simulink model "energy_rigid_wireOnly_quadruped_CPG_BO_fh"  (R2021b)
settings: Solver=ode15s  StartTime=0.0  StopTime=Tf  FixedStep=0.01  MaxStep=0.05  RelTol=0.5  AbsTol=0.5
model workspace (MATLAB code in the model file):
  | %---------------Critical values---------------%
  | angle_amp = pi/4; % Motor rotate amplitude, ref: pi/4
  | rotateCorrectionCoef = 1.158;
  | criticalFn = 2;
  | 
  | %------values for normalization---------------%
  | % values got by running manual gait
  | rotxNormGain = 1/0.1;
  | rotyNormGain = 1/0.05;
  | rotzNormGain = 1/0.1;
  | 
  | vxNormGain = 1/0.2;
  | vyNormGain = 1/0.2;
  | vzNormGain = 1/0.2;
  | 
  | FnNormGain = 1/15;
  | 
  | %--------values for check done---------------%
  | rotDone = pi/6;
  | legBendDone = pi/3; % actuator max bending angle
  | 
  | %---------------Robot parameters-------------%
  | % robot size
  | robot_width = 0.15;
  | robot_length = 0.22;
  | 
  | % floor parameters
  | floor_length = 2;
  | floor_width = 2;
  | 
  | % continuum actuator size
  | L_disk = 0.02944;% Disk side length (m)
  | R_w = L_disk/sqrt(3);
  | thickness_disk = 0.004; % Disk thickness (m)
  | thigh_length = 0.06;
  | R_core = 0.005; % Core radius (m)
  | length_core = 0.008; % Core length (m)
  | R_spool = 0.021; % 0.01944; % radius of the spool
  | spool_height = 0.022+0.015;
  | R_pulley = 1e-3;
  | spool_k = 0;
  | spool_d = 0;
  | hole_d = 4e-3;
  | 
  | % Material property
  | rho_PLA = 1.24e3;
  | rho = 1.19e3; % 1.19e3; % Density (kg/m^3)
  | % use rigid joints
  | Pz_stiff = 135000;
  | Pz_damping = 500*0+2000;
  | S_stiff = 0.0239;
  | S_damping = 7.5e-5;
  | S_low_Bound = -20;
  | S_up_Bound = 20;
  | 
  | R_foot = 0.015; % foot radius (m)
  | 
  | % motor parameter
  | stall_T = 11.2/10; % 11.2 cm*kg, stall torque
  | t_60_deg = 0.2; % 0.09 s
  | V_nomrmal = 6; % corresponding normal voltage
  | Jr = 0.0001; %g*cm^2, robot inertia
  | 
  | % contact force
  | coef_static_friction = 0.315*0+0.6;
  | coef_dynamic_friction = 0.3*0+0.6;
  | crictic_velocity = 0.3; % m/s
  | contact_suf_stiff = 1000*0+750; % N/m
  | contact_suf_damp = 50*0+100; % N/(m/s)
  | contact_region_width = 2e-3; % m
  | spoolOpacity = 0;
  | tendonColor = [0.902 0.902 0.902];
  | tendonOpacity = 0.1;
  | 
  | % If use point masses
  | MMainFrame = 198; % g
  | MServoMotor = 50.55;
  | MMotorSupport = 12.1;
  | MSpool = 9.2;
  | 
  | % Robot total weight about 2 kg
  | MComposateLoad = 200;
  | 
  | MBuck = 40; % x2
  | MPCB_RPi = 141.3;
  | MLiBattery = 120; % x2
  | MPowerBank = 66.5;
  | isLoadVisible = 0.1;
  | 
  | 
  | MThigh = 26.7963;
  | MCore = 0.747699;
  | MDisk = 1.78642;
  | MFoot = 16.8232;
undefined symbols (not defined in the file): A, alpha, alpha_b_gain, alpha_r_gain, DCMotor_K, epsilon, ExtParts, f, init_state, isCheckDone, k, MotorSupport, phase_delay, phi_vec, tau, Tf, TrackStarServo, Ts, WheelCAD, X, Y, Z, z_l_diff, z_l_gain
libraries: sm_lib x311, nesl_utility x81, fl_lib x60, ee_lib x24, slpidlib x12, simulink x11
(part 1 of 16)
settings Model: Creator=Qinglei Ji  LastModifiedBy=kaiget
settings SolverCC: AutoScaleAbsTol=off  MaxConsecutiveZCs=100  MaxConsecutiveMinStep=10  DaesscMode=Fast  ZeroCrossAlgorithm=Adaptive  AutoInsertRateTranBlk=on
settings DebuggingCC: AlgebraicLoopMsg=error  IgnoredZcDiagnostic=none
settings ExplorerConfigSet: InternalSimMechanicsExplorerSettings="<ExplorerConfiguration><canonicalview>default</canonicalview><AnimationSetting><BasePlaybackSpeed>1.0</BasePlaybackSpeed><PlaybackSpeedFactor>1.0</PlaybackSpeedFactor></AnimationSetting><TilePanel><TileInfo><Tiles Columns=\"1\" Count=\"1\" Rows=\"1\"><Column Weight=\"1\"/><Row Weight=\"1\"/><Tile Height=\"1\" Width=\"1\" X=\"0\" Y=\"0\"/></Tiles></TileInfo><SceneInfo><SceneViewer><BGColor><R>0.60000002384185791</R><G>0.60000002384185791</G><B>0.60000002384185791</B></BGColor><Camera><DoPerspective>off</DoPerspective><Position><X>-18.8331461547739707</X><Y>25.880517186070815</Y><Z>26.8100820833696147</Z></Position><Center><X>0.29785977478998571</X><Y>-0.293010908258582892</Y><Z>-0.346783787749327221</Z></Center><Up><X>0.517886432622382209</X><Y>-0.40389178028612327</Y><Z>0.754098848111419029</Z></Up><ViewLimDist>1</ViewLimDist><YLim>0.421333194645766129</YLim><XLim>0.456755011894746488</XLim></Camera></SceneViewer></SceneInfo></TilePanel><MechEditorPanel><Cameras/><GfxPanelCameraMap/><VideoCreator><PlaybackSpeedRatio>1.0</PlaybackSpeedRatio><FrameRate>60</FrameRate><VideoFormat>MPEG-4</VideoFormat><FrameSize>auto</FrameSize></VideoCreator></MechEditorPanel></ExplorerConfiguration>"

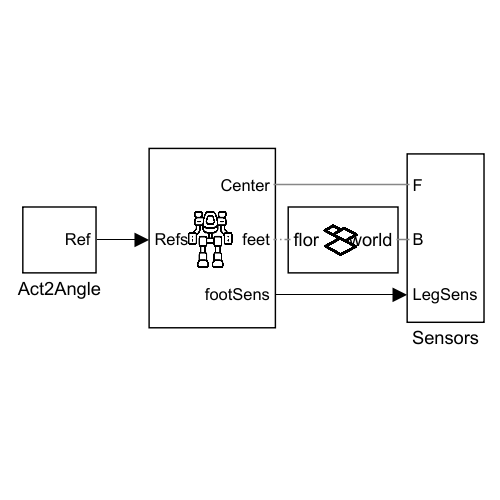
[thumbnail: Simulink's stored preview of the top-level diagram]
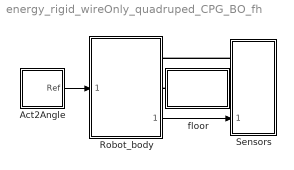
== system energy_rigid_wireOnly_quadruped_CPG_BO_fh ==
  Act2Angle : Subsystem
  Robot_body : Subsystem
      settings: PortSchema="{\"entries\":[{\"content\":{\"sides\":[{\"content\":{\"connectorIds\":[]},\"type\":\"ConnectorPlacement.EquallySpacedRectSide\",\"uuid\":\"6da386a3-61dc-48ac-8951-5f405dad6f0b\"},{\"content\":{\"connectorIds\":[],\"side\":\"RIGHT\"},\"type\":\"ConnectorPlacement.EquallySpacedRectSide\",\"uuid\":\"f31d08fd-e336-4992-a7a1-a5f80310301f\"},{\"content\":{\"connectorIds\":[\"In1\"],\"side\":\"TOP\"},\"type\":\"ConnectorPlacement.EquallySpacedRectSide\",\"uuid\":\"e8d57c74-e878-4fd7-b952-570b3b82c07d\"},{\"content\":{\"connectorIds\":[\"RConn1\",\"RConn2\",\"Out1\"],\"side\":\"BOTTOM\"},\"type\":\"ConnectorPlacement.EquallySpacedRectSide\",\"uuid\":\"5cd044ae-e3eb-4740-b1cb-bb65851cb112\"}]},\"type\":\"ConnectorPlacement.EquallySpacedConnector\",\"uuid\":\"f9915cad-378a-4c2b-ad9c-362eed90ff8c\"}],\"packageUris\":[\"http://schema.mathworks.com/mf0/Connector/R2020b\"],\"version\":\"1.0\"}"
      mask Display: image('$imagefile'); % Use "Edit Image" on toolstrip to change.
  Sensors : Subsystem
      settings: PortSchema="{\"entries\":[{\"content\":{\"sides\":[{\"content\":{\"connectorIds\":[\"LConn1\",\"LConn2\",\"In1\"]},\"type\":\"ConnectorPlacement.EquallySpacedRectSide\",\"uuid\":\"4b5ddd47-03f4-426a-88ee-d6acf531c637\"},{\"content\":{\"connectorIds\":[],\"side\":\"RIGHT\"},\"type\":\"ConnectorPlacement.EquallySpacedRectSide\",\"uuid\":\"f2192e31-fae6-4bce-a663-c668a18a2c9c\"},{\"content\":{\"connectorIds\":[],\"side\":\"TOP\"},\"type\":\"ConnectorPlacement.EquallySpacedRectSide\",\"uuid\":\"20a91eaf-2ad2-4a0d-933a-434c603de7e7\"},{\"content\":{\"connectorIds\":[],\"side\":\"BOTTOM\"},\"type\":\"ConnectorPlacement.EquallySpacedRectSide\",\"uuid\":\"f2757d81-d7c7-43da-8561-08295a517c19\"}]},\"type\":\"ConnectorPlacement.EquallySpacedConnector\",\"uuid\":\"8ce371b8-5669-40c8-963e-855906aef91d\"}],\"packageUris\":[\"http://schema.mathworks.com/mf0/Connector/R2020b\"],\"version\":\"1.0\"}"
  floor : Subsystem
      mask Display: image('$imagefile'); % Use "Edit Image" on toolstrip to change.
  wires:
  Robot_body/1(footSens) -> Sensors/1(LegSens)
  Act2Angle/1(Ref) -> Robot_body/1(motorRefs)
  connections:
  floor/RConn1 -- Robot_body/RConn2
  floor/LConn1 -- Sensors/LConn2
  Sensors/LConn1 -- Robot_body/RConn1

== system energy_rigid_wireOnly_quadruped_CPG_BO_fh/Act2Angle ==
  CPG : Subsystem
  Clock : Clock
  Constant : Constant  Value=zeros(12, 1)
  Human expert : Subsystem  Commented=on
  Manual Switch : ManualSwitch  CurrentSetting=0
  Subsystem : Subsystem
  Switch : Switch  Criteria=u2 > Threshold  Threshold=2
  To Workspace : ToWorkspace  VariableName=action  SaveFormat=Structure  SampleTime=Ts
      settings: Save2DSignal=2-D array (concatenate along first dimension)
  Ref : Outport
  wires:
  Subsystem/1(refs) -> To Workspace/1, Ref/1
  Manual Switch/1 -> Subsystem/1(Acts)  "Acts"
  Human expert/1(Out1) -> Manual Switch/1
  CPG/1(Out2) -> Switch/1
  Clock/1 -> Switch/2
  Constant/1 -> Switch/3
  Switch/1 -> Manual Switch/2

== system energy_rigid_wireOnly_quadruped_CPG_BO_fh/Robot_body ==
  motorRefs : Inport
  6-DOF Joint : sm_lib/Joints/6-DOF Joint  JointMode=Normal  SenseConstraintForce=off  SenseConstraintForceX=off  SenseConstraintForceY=off  SenseConstraintForceZ=off  SenseConstraintTorque=off  SenseConstraintTorqueX=off  SenseConstraintTorqueY=off  SenseConstraintTorqueZ=off  SenseTotalForce=off  SenseTotalForceX=off  SenseTotalForceY=off  SenseTotalForceZ=off  SenseTotalTorque=off  SenseTotalTorqueX=off  SenseTotalTorqueY=off  SenseTotalTorqueZ=off  CompositeWrenchDir=FollowerOnBase  CompositeWrenchFrame=BaseFrame  PxEquilibriumPosition=0  PxEquilibriumPositionUnits=m  PxSpringStiffness=0  PxSpringStiffnessUnits=N/m  PxDampingCoefficient=0  PxDampingCoefficientUnits=N/(m/s)  PxTorqueActuationMode=NoTorque  PxMotionActuationMode=ComputedMotion  PxSensePosition=off  PxSenseVelocity=off  PxSenseAcceleration=off  PxSenseTorqueForce=off  PxSenseLowerLimitTorqueForce=off  PxSenseUpperLimitTorqueForce=off  PxLowerLimitSpecify=off  PxLowerLimitBound=-1  PxLowerLimitBoundUnits=m  PxLowerLimitStiffness=1e6  PxLowerLimitStiffnessUnits=N/m  PxLowerLimitDamping=1e3  PxLowerLimitDampingUnits=N/(m/s)  PxLowerLimitTransitionRegionWidth=1e-4  PxLowerLimitTransitionRegionWidthUnits=m  PxUpperLimitSpecify=off  PxUpperLimitBound=1  PxUpperLimitBoundUnits=m  PxUpperLimitStiffness=1e6  PxUpperLimitStiffnessUnits=N/m  PxUpperLimitDamping=1e3  PxUpperLimitDampingUnits=N/(m/s)  PxUpperLimitTransitionRegionWidth=1e-4  PxUpperLimitTransitionRegionWidthUnits=m  PxPositionTargetSpecify=off  PxPositionTargetPriority=High  PxPositionTargetValue=0  PxPositionTargetValueUnits=m  PxVelocityTargetSpecify=off  PxVelocityTargetPriority=High  PxVelocityTargetValue=0  PxVelocityTargetValueUnits=m/s  PyEquilibriumPosition=0  PyEquilibriumPositionUnits=m  PySpringStiffness=0  PySpringStiffnessUnits=N/m  PyDampingCoefficient=0  PyDampingCoefficientUnits=N/(m/s)  PyTorqueActuationMode=NoTorque  PyMotionActuationMode=ComputedMotion  PySensePosition=off  PySenseVelocity=off  PySenseAcceleration=off  PySenseTorqueForce=off  PySenseLowerLimitTorqueForce=off  PySenseUpperLimitTorqueForce=off  PyLowerLimitSpecify=off  PyLowerLimitBound=-1  PyLowerLimitBoundUnits=m  PyLowerLimitStiffness=1e6  PyLowerLimitStiffnessUnits=N/m  PyLowerLimitDamping=1e3  PyLowerLimitDampingUnits=N/(m/s)  PyLowerLimitTransitionRegionWidth=1e-4  PyLowerLimitTransitionRegionWidthUnits=m  PyUpperLimitSpecify=off  PyUpperLimitBound=1  PyUpperLimitBoundUnits=m  PyUpperLimitStiffness=1e6  PyUpperLimitStiffnessUnits=N/m  PyUpperLimitDamping=1e3  PyUpperLimitDampingUnits=N/(m/s)  PyUpperLimitTransitionRegionWidth=1e-4  PyUpperLimitTransitionRegionWidthUnits=m  PyPositionTargetSpecify=off  PyPositionTargetPriority=High  PyPositionTargetValue=0  PyPositionTargetValueUnits=m  PyVelocityTargetSpecify=off  PyVelocityTargetPriority=High  PyVelocityTargetValue=0  PyVelocityTargetValueUnits=m/s  PzEquilibriumPosition=0  PzEquilibriumPositionUnits=m  PzSpringStiffness=0  PzSpringStiffnessUnits=N/m  PzDampingCoefficient=0  PzDampingCoefficientUnits=N/(m/s)  PzTorqueActuationMode=NoTorque  PzMotionActuationMode=ComputedMotion  PzSensePosition=off  PzSenseVelocity=off  PzSenseAcceleration=off  PzSenseTorqueForce=off  PzSenseLowerLimitTorqueForce=off  PzSenseUpperLimitTorqueForce=off  PzLowerLimitSpecify=off  PzLowerLimitBound=-1  PzLowerLimitBoundUnits=m  PzLowerLimitStiffness=1e6  PzLowerLimitStiffnessUnits=N/m  PzLowerLimitDamping=1e3  PzLowerLimitDampingUnits=N/(m/s)  PzLowerLimitTransitionRegionWidth=1e-4  PzLowerLimitTransitionRegionWidthUnits=m  PzUpperLimitSpecify=off  PzUpperLimitBound=1  PzUpperLimitBoundUnits=m  PzUpperLimitStiffness=1e6  PzUpperLimitStiffnessUnits=N/m  PzUpperLimitDamping=1e3  PzUpperLimitDampingUnits=N/(m/s)  PzUpperLimitTransitionRegionWidth=1e-4  PzUpperLimitTransitionRegionWidthUnits=m  PzPositionTargetSpecify=off  PzPositionTargetPriority=High  PzPositionTargetValue=0  PzPositionTargetValueUnits=m  PzVelocityTargetSpecify=off  PzVelocityTargetPriority=High  PzVelocityTargetValue=0  PzVelocityTargetValueUnits=m/s  SphDefPosRotationMethod=None  SphDefPosRotationAngleUnits=deg  SphDefPosRotationStandardAxis=+Z  SphDefPosRotationAngle=0.0  SphDefPosRotationArbitraryAxis=[0 0 1]  SphDefPosFollAlignAxisA=+X  SphDefPosBaseAlignAxisA=+Y  SphDefPosFollAlignAxisB=+Y  SphDefPosBaseAlignAxisB=+Z  SphDefPosRotationSequenceAxes=FollowerAxes  SphDefPosRotationSequence=XYX  SphDefPosRotationSequenceAngles=[0 0 0]  SphDefPosRotationSequenceAnglesUnits=deg  SphDefPosRotationMatrix=[1 0 0; 0 1 0; 0 0 1]  SphEqPosRotationMethod=None  SphEqPosRotationAngleUnits=deg  SphEqPosRotationStandardAxis=+Z  SphEqPosRotationAngle=0.0  SphEqPosRotationArbitraryAxis=[0 0 1]  SphEqPosFollAlignAxisA=+X  SphEqPosBaseAlignAxisA=+Y  SphEqPosFollAlignAxisB=+Y  SphEqPosBaseAlignAxisB=+Z  SphEqPosRotationSequenceAxes=FollowerAxes  SphEqPosRotationSequence=XYX  SphEqPosRotationSequenceAngles=[0 0 0]  SphEqPosRotationSequenceAnglesUnits=deg  SphEqPosRotationMatrix=[1 0 0; 0 1 0; 0 0 1]  SphSpringStiffness=0  SphSpringStiffnessUnits=N*m/deg  SphDampingCoefficient=0  SphDampingCoefficientUnits=N*m/(deg/s)  SphActuateTorqueX=off  SphActuateTorqueY=off  SphActuateTorqueZ=off  SphActuateTorque=off  SphTorqueActuationMode=NoTorque  SphMotionActuationMode=ComputedMotion  SphActuationFrame=BaseFrame  SphSensePosition=off  SphSenseVelocityX=off  SphSenseVelocityY=off  SphSenseVelocityZ=off  SphSenseVelocity=off  SphSenseAccelerationX=off  SphSenseAccelerationY=off  SphSenseAccelerationZ=off  SphSenseAcceleration=off  SphSenseTorqueX=off  SphSenseTorqueY=off  SphSenseTorqueZ=off  SphSenseTorqueForce=off  SphSenseLowerLimitTorqueMag=off  SphSenseUpperLimitTorqueMag=off  SphSensingFrame=BaseFrame  SphLowerLimitSpecify=off  SphLowerLimitBound=15  SphLowerLimitBoundUnits=deg  SphLowerLimitStiffness=1e4  SphLowerLimitStiffnessUnits=N*m/deg  SphLowerLimitDamping=10  SphLowerLimitDampingUnits=N*m/(deg/s)  SphLowerLimitTransitionRegionWidth=0.1  SphLowerLimitTransitionRegionWidthUnits=deg  SphUpperLimitSpecify=off  SphUpperLimitBound=45  SphUpperLimitBoundUnits=deg  SphUpperLimitStiffness=1e4  SphUpperLimitStiffnessUnits=N*m/deg  SphUpperLimitDamping=10  SphUpperLimitDampingUnits=N*m/(deg/s)  SphUpperLimitTransitionRegionWidth=0.1  SphUpperLimitTransitionRegionWidthUnits=deg  SphPositionTargetRotationMethod=None  SphPositionTargetRotationAngleUnits=deg  SphPositionTargetRotationStandardAxis=+Z  SphPositionTargetRotationAngle=0.0  SphPositionTargetRotationArbitraryAxis=[0 0 1]  SphPositionTargetFollAlignAxisA=+X  SphPositionTargetBaseAlignAxisA=+Y  SphPositionTargetFollAlignAxisB=+Y  SphPositionTargetBaseAlignAxisB=+Z  SphPositionTargetRotationSequenceAxes=FollowerAxes  SphPositionTargetRotationSequence=XYX  SphPositionTargetRotationSequenceAngles=[0 0 0]  SphPositionTargetRotationSequenceAnglesUnits=deg  SphPositionTargetRotationMatrix=[1 0 0; 0 1 0; 0 0 1]  SphPositionTargetSpecify=off  SphPositionTargetPriority=High  SphVelocityTargetValue=[0 0 0]  SphVelocityTargetValueUnits=deg/s  SphVelocityTargetSpecify=off  SphVelocityTargetPriority=High  SphVelocityTargetInFollowerFrame=on
  Bus Creator : BusCreator  Inputs=12
  Demux : Demux
  FL : Subsystem
  FR : Subsystem
  FootFL : Subsystem
      settings: PortSchema="{\"entries\":[{\"content\":{\"sides\":[{\"content\":{\"connectorIds\":[\"LConn1\",\"Out1\"]},\"type\":\"ConnectorPlacement.EquallySpacedRectSide\",\"uuid\":\"0bb1f20c-4b5e-487a-8abf-3e1f2fef015b\"},{\"content\":{\"connectorIds\":[\"RConn1\"],\"side\":\"RIGHT\"},\"type\":\"ConnectorPlacement.EquallySpacedRectSide\",\"uuid\":\"5d13e6ab-8a90-4d8e-960d-d3cf2c1ae97d\"},{\"content\":{\"connectorIds\":[],\"side\":\"TOP\"},\"type\":\"ConnectorPlacement.EquallySpacedRectSide\",\"uuid\":\"95bd9573-7fea-4bcb-a448-c8ab92610e8b\"},{\"content\":{\"connectorIds\":[],\"side\":\"BOTTOM\"},\"type\":\"ConnectorPlacement.EquallySpacedRectSide\",\"uuid\":\"976c40b0-0fd4-4a26-8e09-25e540e36d50\"}]},\"type\":\"ConnectorPlacement.EquallySpacedConnector\",\"uuid\":\"5d9c26bf-393c-4096-afaf-0ed92cf9ce69\"}],\"packageUris\":[\"http://schema.mathworks.com/mf0/Connector/R2020b\"],\"version\":\"1.0\"}"
  FootFR : Subsystem
      settings: PortSchema="{\"entries\":[{\"content\":{\"sides\":[{\"content\":{\"connectorIds\":[\"LConn1\",\"Out1\"]},\"type\":\"ConnectorPlacement.EquallySpacedRectSide\",\"uuid\":\"0bb1f20c-4b5e-487a-8abf-3e1f2fef015b\"},{\"content\":{\"connectorIds\":[\"RConn1\"],\"side\":\"RIGHT\"},\"type\":\"ConnectorPlacement.EquallySpacedRectSide\",\"uuid\":\"5d13e6ab-8a90-4d8e-960d-d3cf2c1ae97d\"},{\"content\":{\"connectorIds\":[],\"side\":\"TOP\"},\"type\":\"ConnectorPlacement.EquallySpacedRectSide\",\"uuid\":\"95bd9573-7fea-4bcb-a448-c8ab92610e8b\"},{\"content\":{\"connectorIds\":[],\"side\":\"BOTTOM\"},\"type\":\"ConnectorPlacement.EquallySpacedRectSide\",\"uuid\":\"976c40b0-0fd4-4a26-8e09-25e540e36d50\"}]},\"type\":\"ConnectorPlacement.EquallySpacedConnector\",\"uuid\":\"5d9c26bf-393c-4096-afaf-0ed92cf9ce69\"}],\"packageUris\":[\"http://schema.mathworks.com/mf0/Connector/R2020b\"],\"version\":\"1.0\"}"
  FootRL : Subsystem
      settings: PortSchema="{\"entries\":[{\"content\":{\"sides\":[{\"content\":{\"connectorIds\":[\"LConn1\",\"Out1\"]},\"type\":\"ConnectorPlacement.EquallySpacedRectSide\",\"uuid\":\"0bb1f20c-4b5e-487a-8abf-3e1f2fef015b\"},{\"content\":{\"connectorIds\":[\"RConn1\"],\"side\":\"RIGHT\"},\"type\":\"ConnectorPlacement.EquallySpacedRectSide\",\"uuid\":\"5d13e6ab-8a90-4d8e-960d-d3cf2c1ae97d\"},{\"content\":{\"connectorIds\":[],\"side\":\"TOP\"},\"type\":\"ConnectorPlacement.EquallySpacedRectSide\",\"uuid\":\"95bd9573-7fea-4bcb-a448-c8ab92610e8b\"},{\"content\":{\"connectorIds\":[],\"side\":\"BOTTOM\"},\"type\":\"ConnectorPlacement.EquallySpacedRectSide\",\"uuid\":\"976c40b0-0fd4-4a26-8e09-25e540e36d50\"}]},\"type\":\"ConnectorPlacement.EquallySpacedConnector\",\"uuid\":\"5d9c26bf-393c-4096-afaf-0ed92cf9ce69\"}],\"packageUris\":[\"http://schema.mathworks.com/mf0/Connector/R2020b\"],\"version\":\"1.0\"}"
  FootRR : Subsystem
      settings: PortSchema="{\"entries\":[{\"content\":{\"sides\":[{\"content\":{\"connectorIds\":[\"LConn1\",\"Out1\"]},\"type\":\"ConnectorPlacement.EquallySpacedRectSide\",\"uuid\":\"0bb1f20c-4b5e-487a-8abf-3e1f2fef015b\"},{\"content\":{\"connectorIds\":[\"RConn1\"],\"side\":\"RIGHT\"},\"type\":\"ConnectorPlacement.EquallySpacedRectSide\",\"uuid\":\"5d13e6ab-8a90-4d8e-960d-d3cf2c1ae97d\"},{\"content\":{\"connectorIds\":[],\"side\":\"TOP\"},\"type\":\"ConnectorPlacement.EquallySpacedRectSide\",\"uuid\":\"95bd9573-7fea-4bcb-a448-c8ab92610e8b\"},{\"content\":{\"connectorIds\":[],\"side\":\"BOTTOM\"},\"type\":\"ConnectorPlacement.EquallySpacedRectSide\",\"uuid\":\"976c40b0-0fd4-4a26-8e09-25e540e36d50\"}]},\"type\":\"ConnectorPlacement.EquallySpacedConnector\",\"uuid\":\"5d9c26bf-393c-4096-afaf-0ed92cf9ce69\"}],\"packageUris\":[\"http://schema.mathworks.com/mf0/Connector/R2020b\"],\"version\":\"1.0\"}"
  RL : Subsystem
  RR : Subsystem
  Rigid Transform : sm_lib/Frames and Transforms/Rigid Transform  TranslationMethod=None  TranslationStandardOffset=0.1  TranslationLengthUnit=m  TranslationStandardAxis=+Z  TranslationCartesianOffset=[0 0 0]  TranslationROffset=0  TranslationROffsetUnits=m  TranslationZOffset=0  TranslationZOffsetUnits=m  TranslationThetaOffset=0  TranslationThetaOffsetUnits=deg  RotationMethod=StandardAxis  RotationAngleUnits=deg  RotationStandardAxis=-Z  RotationAngle=90  RotationArbitraryAxis=[0 0 1]  FollAlignAxisA=+X  BaseAlignAxisA=+Z  FollAlignAxisB=+Y  BaseAlignAxisB=+Z  RotationSequenceAxes=FollowerAxes  RotationSequence=XYX  RotationSequenceAngles=[0 0 0]  RotationSequenceAnglesUnits=deg  RotationMatrix=[1 0 0; 0 1 0; 0 0 1]
  Rigid Transform1 : sm_lib/Frames and Transforms/Rigid Transform  TranslationMethod=None  TranslationStandardOffset=0.1  TranslationLengthUnit=m  TranslationStandardAxis=+Z  TranslationCartesianOffset=[0 0 0]  TranslationROffset=0  TranslationROffsetUnits=m  TranslationZOffset=0  TranslationZOffsetUnits=m  TranslationThetaOffset=0  TranslationThetaOffsetUnits=deg  RotationMethod=StandardAxis  RotationAngleUnits=deg  RotationStandardAxis=+Z  RotationAngle=90  RotationArbitraryAxis=[0 0 1]  FollAlignAxisA=+X  BaseAlignAxisA=+Z  FollAlignAxisB=+Y  BaseAlignAxisB=+Z  RotationSequenceAxes=FollowerAxes  RotationSequence=XYX  RotationSequenceAngles=[0 0 0]  RotationSequenceAnglesUnits=deg  RotationMatrix=[1 0 0; 0 1 0; 0 0 1]
  Rigid Transform2 : sm_lib/Frames and Transforms/Rigid Transform  TranslationMethod=Cartesian  TranslationStandardOffset=0  TranslationLengthUnit=m  TranslationStandardAxis=+Z  TranslationCartesianOffset=[robot_length/2 -robot_width/2 0]  TranslationROffset=0  TranslationROffsetUnits=m  TranslationZOffset=0  TranslationZOffsetUnits=m  TranslationThetaOffset=0  TranslationThetaOffsetUnits=deg  RotationMethod=None  RotationAngleUnits=deg  RotationStandardAxis=+Z  RotationAngle=0.0  RotationArbitraryAxis=[0 0 1]  FollAlignAxisA=+X  BaseAlignAxisA=+Y  FollAlignAxisB=+Y  BaseAlignAxisB=+Z  RotationSequenceAxes=FollowerAxes  RotationSequence=XYX  RotationSequenceAngles=[0 0 0]  RotationSequenceAnglesUnits=deg  RotationMatrix=[1 0 0; 0 1 0; 0 0 1]
  Rigid Transform3 : sm_lib/Frames and Transforms/Rigid Transform  TranslationMethod=Cartesian  TranslationStandardOffset=0  TranslationLengthUnit=m  TranslationStandardAxis=+Z  TranslationCartesianOffset=[robot_length/2 robot_width/2 0]  TranslationROffset=0  TranslationROffsetUnits=m  TranslationZOffset=0  TranslationZOffsetUnits=m  TranslationThetaOffset=0  TranslationThetaOffsetUnits=deg  RotationMethod=None  RotationAngleUnits=deg  RotationStandardAxis=+Z  RotationAngle=0.0  RotationArbitraryAxis=[0 0 1]  FollAlignAxisA=+X  BaseAlignAxisA=+Y  FollAlignAxisB=+Y  BaseAlignAxisB=+Z  RotationSequenceAxes=FollowerAxes  RotationSequence=XYX  RotationSequenceAngles=[0 0 0]  RotationSequenceAnglesUnits=deg  RotationMatrix=[1 0 0; 0 1 0; 0 0 1]
  Rigid Transform4 : sm_lib/Frames and Transforms/Rigid Transform  TranslationMethod=Cartesian  TranslationStandardOffset=0  TranslationLengthUnit=m  TranslationStandardAxis=+Z  TranslationCartesianOffset=[-robot_length/2 -robot_width/2 0]  TranslationROffset=0  TranslationROffsetUnits=m  TranslationZOffset=0  TranslationZOffsetUnits=m  TranslationThetaOffset=0  TranslationThetaOffsetUnits=deg  RotationMethod=None  RotationAngleUnits=deg  RotationStandardAxis=+Z  RotationAngle=0.0  RotationArbitraryAxis=[0 0 1]  FollAlignAxisA=+X  BaseAlignAxisA=+Y  FollAlignAxisB=+Y  BaseAlignAxisB=+Z  RotationSequenceAxes=FollowerAxes  RotationSequence=XYX  RotationSequenceAngles=[0 0 0]  RotationSequenceAnglesUnits=deg  RotationMatrix=[1 0 0; 0 1 0; 0 0 1]
  Rigid Transform5 : sm_lib/Frames and Transforms/Rigid Transform  TranslationMethod=Cartesian  TranslationStandardOffset=0  TranslationLengthUnit=m  TranslationStandardAxis=+Z  TranslationCartesianOffset=[-robot_length/2 robot_width/2 0]  TranslationROffset=0  TranslationROffsetUnits=m  TranslationZOffset=0  TranslationZOffsetUnits=m  TranslationThetaOffset=0  TranslationThetaOffsetUnits=deg  RotationMethod=None  RotationAngleUnits=deg  RotationStandardAxis=+Z  RotationAngle=0.0  RotationArbitraryAxis=[0 0 1]  FollAlignAxisA=+X  BaseAlignAxisA=+Y  FollAlignAxisB=+Y  BaseAlignAxisB=+Z  RotationSequenceAxes=FollowerAxes  RotationSequence=XYX  RotationSequenceAngles=[0 0 0]  RotationSequenceAnglesUnits=deg  RotationMatrix=[1 0 0; 0 1 0; 0 0 1]
  Rigid Transform9 : sm_lib/Frames and Transforms/Rigid Transform  TranslationMethod=Cartesian  TranslationStandardOffset=0  TranslationLengthUnit=m  TranslationStandardAxis=+Z  TranslationCartesianOffset=[0 0 0.155]  TranslationROffset=0  TranslationROffsetUnits=m  TranslationZOffset=0  TranslationZOffsetUnits=m  TranslationThetaOffset=0  TranslationThetaOffsetUnits=deg  RotationMethod=StandardAxis  RotationAngleUnits=deg  RotationStandardAxis=+Y  RotationAngle=0  RotationArbitraryAxis=[0 0 1]  FollAlignAxisA=+X  BaseAlignAxisA=+Y  FollAlignAxisB=+Y  BaseAlignAxisB=+Z  RotationSequenceAxes=FollowerAxes  RotationSequence=XYX  RotationSequenceAngles=[0 0 0]  RotationSequenceAnglesUnits=deg  RotationMatrix=[1 0 0; 0 1 0; 0 0 1]
  StructureDisk : Subsystem
      settings: PortSchema="{\"entries\":[{\"content\":{\"sides\":[{\"content\":{\"connectorIds\":[]},\"type\":\"ConnectorPlacement.EquallySpacedRectSide\",\"uuid\":\"983b4593-33f8-4f05-8496-f6a680e0506a\"},{\"content\":{\"connectorIds\":[\"RConn1\"],\"side\":\"RIGHT\"},\"type\":\"ConnectorPlacement.EquallySpacedRectSide\",\"uuid\":\"dd1cb835-99ed-40eb-9457-9a76e9b19610\"},{\"content\":{\"connectorIds\":[\"LConn1\"],\"side\":\"TOP\"},\"type\":\"ConnectorPlacement.EquallySpacedRectSide\",\"uuid\":\"c15c4885-45e6-4882-9e3a-df9802ff439f\"}]},\"type\":\"ConnectorPlacement.EquallySpacedConnector\",\"uuid\":\"19826241-0a68-4e2d-83d2-fcb027292ea7\"}],\"packageUris\":[\"http://schema.mathworks.com/mf0/Connector/R2020b\"],\"version\":\"1.0\"}"
      mask DialogControl DescTextVar Prompt: StructureDisk.png
      mask Display: image('$imagefile'); % Use "Edit Image" on toolstrip to change.
  World Frame : sm_lib/Frames and Transforms/World Frame
  sensFL : Subsystem
      settings: PortSchema="{\"entries\":[{\"content\":{\"sides\":[{\"content\":{\"connectorIds\":[]},\"type\":\"ConnectorPlacement.EquallySpacedRectSide\",\"uuid\":\"bd83465d-2bef-45ec-b31a-ccd96dc04922\"},{\"content\":{\"connectorIds\":[],\"side\":\"RIGHT\"},\"type\":\"ConnectorPlacement.EquallySpacedRectSide\",\"uuid\":\"7d39c37e-7359-45a9-8850-f640f6442332\"},{\"content\":{\"connectorIds\":[\"LConn1\"],\"side\":\"TOP\"},\"type\":\"ConnectorPlacement.EquallySpacedRectSide\",\"uuid\":\"9171d6ae-b8cc-4ed2-b32d-fb0addba6640\"},{\"content\":{\"connectorIds\":[\"Out1\",\"RConn1\"],\"side\":\"BOTTOM\"},\"type\":\"ConnectorPlacement.EquallySpacedRectSide\",\"uuid\":\"6d61618f-1cbe-4c91-8d9a-cf1c63ddd154\"}]},\"type\":\"ConnectorPlacement.EquallySpacedConnector\",\"uuid\":\"3aecd3e6-ec94-4a95-ad20-92352af1806b\"}],\"packageUris\":[\"http://schema.mathworks.com/mf0/Connector/R2020b\"],\"version\":\"1.0\"}"
  sensFR : Subsystem
      settings: PortSchema="{\"entries\":[{\"content\":{\"sides\":[{\"content\":{\"connectorIds\":[]},\"type\":\"ConnectorPlacement.EquallySpacedRectSide\",\"uuid\":\"bd83465d-2bef-45ec-b31a-ccd96dc04922\"},{\"content\":{\"connectorIds\":[],\"side\":\"RIGHT\"},\"type\":\"ConnectorPlacement.EquallySpacedRectSide\",\"uuid\":\"7d39c37e-7359-45a9-8850-f640f6442332\"},{\"content\":{\"connectorIds\":[\"LConn1\"],\"side\":\"TOP\"},\"type\":\"ConnectorPlacement.EquallySpacedRectSide\",\"uuid\":\"9171d6ae-b8cc-4ed2-b32d-fb0addba6640\"},{\"content\":{\"connectorIds\":[\"Out1\",\"RConn1\"],\"side\":\"BOTTOM\"},\"type\":\"ConnectorPlacement.EquallySpacedRectSide\",\"uuid\":\"6d61618f-1cbe-4c91-8d9a-cf1c63ddd154\"}]},\"type\":\"ConnectorPlacement.EquallySpacedConnector\",\"uuid\":\"3aecd3e6-ec94-4a95-ad20-92352af1806b\"}],\"packageUris\":[\"http://schema.mathworks.com/mf0/Connector/R2020b\"],\"version\":\"1.0\"}"
  sensRL : Subsystem
      settings: PortSchema="{\"entries\":[{\"content\":{\"sides\":[{\"content\":{\"connectorIds\":[]},\"type\":\"ConnectorPlacement.EquallySpacedRectSide\",\"uuid\":\"bd83465d-2bef-45ec-b31a-ccd96dc04922\"},{\"content\":{\"connectorIds\":[],\"side\":\"RIGHT\"},\"type\":\"ConnectorPlacement.EquallySpacedRectSide\",\"uuid\":\"7d39c37e-7359-45a9-8850-f640f6442332\"},{\"content\":{\"connectorIds\":[\"LConn1\"],\"side\":\"TOP\"},\"type\":\"ConnectorPlacement.EquallySpacedRectSide\",\"uuid\":\"9171d6ae-b8cc-4ed2-b32d-fb0addba6640\"},{\"content\":{\"connectorIds\":[\"Out1\",\"RConn1\"],\"side\":\"BOTTOM\"},\"type\":\"ConnectorPlacement.EquallySpacedRectSide\",\"uuid\":\"6d61618f-1cbe-4c91-8d9a-cf1c63ddd154\"}]},\"type\":\"ConnectorPlacement.EquallySpacedConnector\",\"uuid\":\"3aecd3e6-ec94-4a95-ad20-92352af1806b\"}],\"packageUris\":[\"http://schema.mathworks.com/mf0/Connector/R2020b\"],\"version\":\"1.0\"}"
  sensRR : Subsystem
      settings: PortSchema="{\"entries\":[{\"content\":{\"sides\":[{\"content\":{\"connectorIds\":[]},\"type\":\"ConnectorPlacement.EquallySpacedRectSide\",\"uuid\":\"bd83465d-2bef-45ec-b31a-ccd96dc04922\"},{\"content\":{\"connectorIds\":[],\"side\":\"RIGHT\"},\"type\":\"ConnectorPlacement.EquallySpacedRectSide\",\"uuid\":\"7d39c37e-7359-45a9-8850-f640f6442332\"},{\"content\":{\"connectorIds\":[\"LConn1\"],\"side\":\"TOP\"},\"type\":\"ConnectorPlacement.EquallySpacedRectSide\",\"uuid\":\"9171d6ae-b8cc-4ed2-b32d-fb0addba6640\"},{\"content\":{\"connectorIds\":[\"Out1\",\"RConn1\"],\"side\":\"BOTTOM\"},\"type\":\"ConnectorPlacement.EquallySpacedRectSide\",\"uuid\":\"6d61618f-1cbe-4c91-8d9a-cf1c63ddd154\"}]},\"type\":\"ConnectorPlacement.EquallySpacedConnector\",\"uuid\":\"3aecd3e6-ec94-4a95-ad20-92352af1806b\"}],\"packageUris\":[\"http://schema.mathworks.com/mf0/Connector/R2020b\"],\"version\":\"1.0\"}"
  Center : PMIOPort  Side=Right
  feet : PMIOPort  Port=2  Side=Right
  footSens : Outport
  wires:
  [refFR] -> FR/1(In1)  "refFR"
  [refFL] -> FL/1(In1)  "refFL"
  [refRR] -> RR/1(In1)  "refRR"
  [refRL] -> RL/1(In1)  "refRL"
  Bus Creator/1 -> footSens/1
  FootFR/1(sensor) -> Bus Creator/2
  FootFL/1(sensor) -> Bus Creator/5
  FootRL/1(sensor) -> Bus Creator/8
  FootRR/1(sensor) -> Bus Creator/11
  sensFR/1(bend) -> Bus Creator/3
  sensFL/1(bend) -> Bus Creator/6
  sensRL/1(bend) -> Bus Creator/9
  sensRR/1(bend) -> Bus Creator/12
  Demux/1 -> [refFR]
  Demux/2 -> [refFL]
  Demux/3 -> [refRL]
  Demux/4 -> [refRR]
  motorRefs/1 -> Demux/1  "Refs"
  FR/1(powers) -> Bus Creator/1  "powerFR"
  FL/1(powers) -> Bus Creator/4  "powerFL"
  RL/1(powers) -> Bus Creator/7  "powerRL"
  RR/1(powers) -> Bus Creator/10  "powerRR"
  connections:
  sensFL/LConn1 -- FL/LConn1 -- Rigid Transform4/LConn1
  sensRR/LConn1 -- RR/LConn1 -- Rigid Transform3/LConn1
  sensRL/LConn1 -- RL/LConn1 -- Rigid Transform2/LConn1
  FootFR/LConn1 -- FootFL/LConn1 -- feet/RConn1 -- FootRR/LConn1 -- FootRL/LConn1
  sensFL/RConn1 -- FL/RConn1 -- FootFL/RConn1
  sensRL/RConn1 -- RL/RConn1 -- FootRL/RConn1
  sensRR/RConn1 -- RR/RConn1 -- FootRR/RConn1
  Rigid Transform2/RConn1 -- Rigid Transform3/RConn1 -- Rigid Transform1/LConn1 -- Rigid Transform5/RConn1 -- Rigid Transform4/RConn1
  Rigid Transform/LConn1 -- StructureDisk/LConn1
  StructureDisk/RConn1 -- Rigid Transform1/RConn1
  Rigid Transform/RConn1 -- 6-DOF Joint/RConn1 -- Center/RConn1
  FR/LConn1 -- sensFR/LConn1 -- Rigid Transform5/LConn1
  FR/RConn1 -- FootFR/RConn1 -- sensFR/RConn1
  Rigid Transform9/RConn1 -- 6-DOF Joint/LConn1
  Rigid Transform9/LConn1 -- World Frame/RConn1

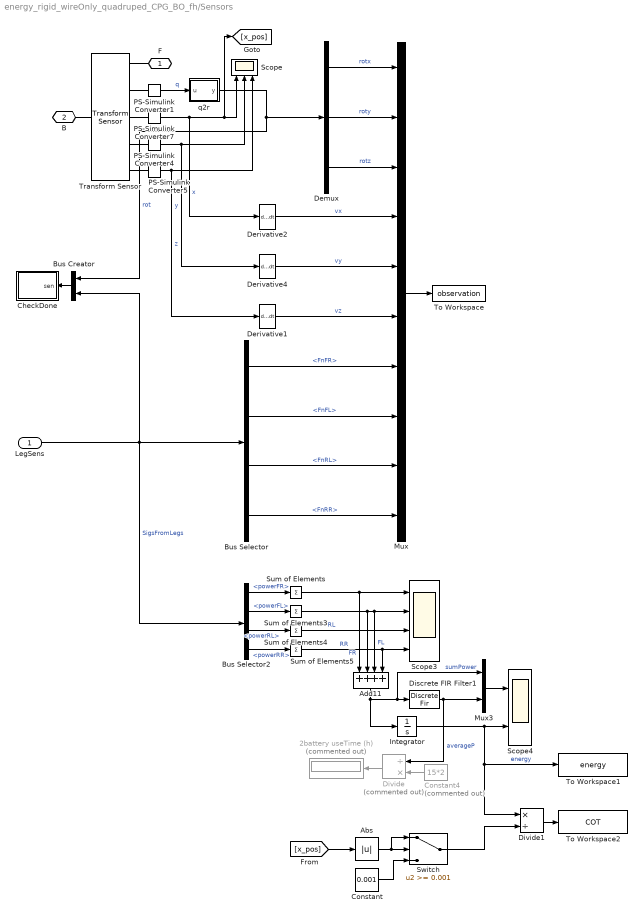
== system energy_rigid_wireOnly_quadruped_CPG_BO_fh/Sensors ==
  LegSens : Inport
  2battery useTime (h) : Display  Commented=on
  Abs : Abs
  Add11 : Sum  Inputs=++++
  Bus Creator : BusCreator  Inputs=2
  Bus Selector : BusSelector  OutputSignals=FnFR,FnFL,FnRL,FnRR
  Bus Selector2 : BusSelector  OutputSignals=powerFR,powerFL,powerRL,powerRR
  CheckDone : Subsystem
  Constant : Constant  Value=0.001
  Constant4 : Constant  Commented=on  Value=15*2
  Demux : Demux  Outputs=3
  Derivative1 : Derivative
  Derivative2 : Derivative
  Derivative4 : Derivative
  Discrete FIR Filter1 : DiscreteFir  Coefficients=ones(1,20)/20
  Divide : Product  Commented=on  Inputs=/*
  Divide1 : Product  Inputs=*/
  Integrator : Integrator
  Mux : Mux  Inputs=10
  Mux3 : Mux  Inputs=2
  PS-Simulink Converter{1,4..5,7} (4 alike) : nesl_utility/PS-Simulink Converter  PhysicalDomain=network_engine_domain  SubClassName=ps_output  LeftPortType=input  RightPortType=output  PseudoPeriodic=off  Frequencies=[]  Unit=1  AffineConversion=off
      settings: SourceProductBaseCode=PW,SS
  Scope : Scope  NumInputPorts=3
  Scope3 : Scope  NumInputPorts=4
  Scope4 : Scope  NumInputPorts=2
  Sum of Elements{,3..5} (4 alike) : Sum  Inputs=+
  Switch : Switch  Threshold=0.001
  To Workspace : ToWorkspace  VariableName=observation  SaveFormat=Structure  SampleTime=Ts
      settings: Save2DSignal=2-D array (concatenate along first dimension)
  To Workspace1 : ToWorkspace  VariableName=energy  SaveFormat=Timeseries  SampleTime=Ts
      settings: Save2DSignal=2-D array (concatenate along first dimension)
  To Workspace2 : ToWorkspace  VariableName=COT  SaveFormat=Timeseries  SampleTime=Ts
      settings: Save2DSignal=2-D array (concatenate along first dimension)
  Transform Sensor : sm_lib/Frames and Transforms/Transform Sensor  MeasurementFrame=World  SenseAngle=off  SenseAxis=off  SenseAngle1=off  SenseAngle2=off  SenseAngle3=off  SenseQ=on  SenseR=off  SenseOmegaX=off  SenseOmegaY=off  SenseOmegaZ=off  SenseOmega1=off  SenseOmega2=off  SenseOmega3=off  SenseQDot=off  SenseRDot=off  SenseAlphaX=off  SenseAlphaY=off  SenseAlphaZ=off  SenseAlpha1=off  SenseAlpha2=off  SenseAlpha3=off  SenseQDDot=off  SenseRDDot=off  SenseX=on  SenseY=on  SenseZ=on  SenseRad=off  SenseAzim=off  SenseDist=off  SenseInc=off  SenseXDot=off  SenseYDot=off  SenseZDot=off  SenseRadDot=off  SenseAzimDot=off  SenseDistDot=off  SenseIncDot=off  SenseXDDot=off  SenseYDDot=off  SenseZDDot=off  SenseRadDDot=off  SenseAzimDDot=off  SenseDistDDot=off  SenseIncDDot=off
  q2r : MATLAB Function  TreatAsAtomicUnit=on
  F : PMIOPort  Side=Left
  B : PMIOPort  Port=2  Side=Left
  wires:
  PS-Simulink Converter1/1 -> q2r/1(u)  "q"
  PS-Simulink Converter5/1 -> Derivative1/1, Scope/3  "z"
  Derivative2/1 -> Mux/4  "vx"
  Derivative4/1 -> Mux/5  "vy"
  Derivative1/1 -> Mux/6  "vz"
  PS-Simulink Converter4/1 -> Scope/2, Derivative4/1  "y"
  PS-Simulink Converter7/1 -> Derivative2/1, [x_pos], Scope/1  "x"
  Mux/1 -> To Workspace/1
  q2r/1(y) -> Bus Creator/1, Demux/1  "rot"
  Demux/1 -> Mux/1  "rotx"
  Demux/2 -> Mux/2  "roty"
  Demux/3 -> Mux/3  "rotz"
  LegSens/1 -> Bus Selector2/1, Bus Selector/1, Bus Creator/2  "SigsFromLegs"
  Bus Selector/1 -> Mux/7  "<FnFR>"
  Bus Selector/2 -> Mux/8  "<FnFL>"
  Bus Selector/3 -> Mux/9  "<FnRL>"
  Bus Selector/4 -> Mux/10  "<FnRR>"
  Bus Creator/1 -> CheckDone/1(sen)
  Constant4/1 -> Divide/2
  Add11/1 -> Integrator/1, Discrete FIR Filter1/1, Mux3/1  "sumPower"
  Mux3/1 -> Scope4/1
  Sum of Elements4/1 -> Scope3/3  "RL"
  Integrator/1 -> Scope4/2, Divide1/1, To Workspace1/1  "energy"
  Bus Selector2/3 -> Sum of Elements4/1  "<powerRL>"
  Bus Selector2/1 -> Sum of Elements/1  "<powerFR>"
  Bus Selector2/2 -> Sum of Elements3/1  "<powerFL>"
  Sum of Elements3/1 -> Add11/2, Add11/3, Scope3/2  "FL"
  Sum of Elements5/1 -> Add11/4, Scope3/4  "RR"
  Bus Selector2/4 -> Sum of Elements5/1  "<powerRR>"
  Sum of Elements/1 -> Add11/1, Scope3/1  "FR"
  Divide/1 -> 2battery useTime (h)/1
  Discrete FIR Filter1/1 -> Mux3/2, Divide/1  "averageP"
  [x_pos] -> Abs/1
  Divide1/1 -> To Workspace2/1
  Abs/1 -> Switch/1, Switch/2
  Constant/1 -> Switch/3
  Switch/1 -> Divide1/2
  connections:
  F/RConn1 -- Transform Sensor/RConn1
  B/RConn1 -- Transform Sensor/LConn1
  PS-Simulink Converter1/LConn1 -- Transform Sensor/RConn2
  Transform Sensor/RConn3 -- PS-Simulink Converter7/LConn1
  PS-Simulink Converter4/LConn1 -- Transform Sensor/RConn4
  PS-Simulink Converter5/LConn1 -- Transform Sensor/RConn5

== system energy_rigid_wireOnly_quadruped_CPG_BO_fh/floor ==
  Grid Plane : Subsystem  Description=Grid block, GA, 2021  mask(Grid Block){length=floor_length, width=floor_width, numSqrs=2, lineWidth=0.005, gridColor=[0.6 0.6 0.6], gridOpacity=0.7, planeColor=[0.8 1.0 1.0], planeOpacity=1}
      mask prompts: length "Length (m)"; width "Width (m)"; numSqrs "Number of Squares"; lineWidth "Line Width (m)"; gridColor "Grid Color [R G B]"; gridOpacity "Grid Opacity"; planeColor "Plane Color [R G B]"; planeOpacity "Plane Opacity"
      mask help:
      | This block creates a grid plane using the Extr_Data_Mesh() function included in the "Simscape Multibody Parts Library" add-on. Please make sure that you have that add-on installed before using this block.
      | Georgios Andrikopoulos, KTH, 2021
      mask init:
      | box_h = (length - ...
      |     (lineWidth*(numSqrs+1)))/...
      |     numSqrs;
      | box_l = (length - ...
      |     (lineWidth*(1+1)))/1;
      | layer1 = Extr_Data_Mesh(width,...
      |     width,numSqrs,1,...
      |     box_h,box_l);
      | 
      | box_h2 = (length - ...
      |     ((lineWidth/3)*((numSqrs*10)+1)))/...
      |     (numSqrs*10);
      | box_l2 = (length - ...
      |     ((lineWidth/3)*(1+1)))/1;
      | layer2 = Extr_Data_Mesh(width,...
      |     width,(numSqrs*10),1,...
      |     box_h2,box_l2);
      | 
      | box_h3 = (length - ...
      |     ((lineWidth/20)*((numSqrs*100)+1)))/...
      |     (numSqrs*100);
      | box_l3 = (length - ...
      |     ((lineWidth/20)*(1+1)))/1;
      | layer3 = Extr_Data_Mesh(width,...
      |     width,(numSqrs*100),1,...
      |     box_h3,box_l3);
  worldSetting : Subsystem
  world : PMIOPort  Side=Left
  flor : PMIOPort  Port=2  Side=Right
  connections:
  Grid Plane/RConn1 -- flor/RConn1
  world/RConn1 -- Grid Plane/LConn1 -- worldSetting/RConn1

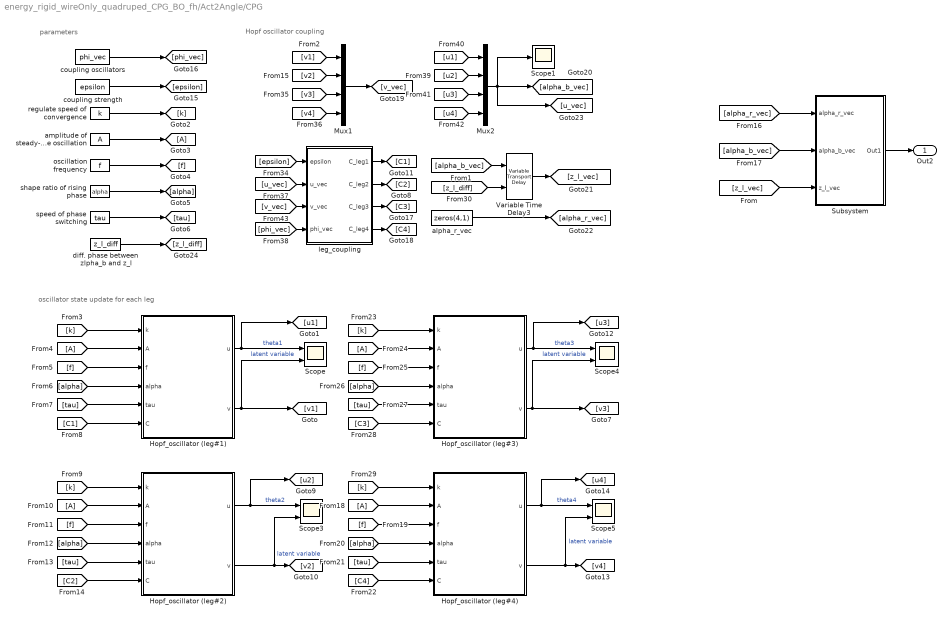
== system energy_rigid_wireOnly_quadruped_CPG_BO_fh/Act2Angle/CPG ==
  note: oscillator state update for each leg
  note: Hopf oscillator coupling
  note: parameters
  Hopf_oscillator (leg#1) : Subsystem
  Hopf_oscillator (leg#2) : Subsystem
  Hopf_oscillator (leg#3) : Subsystem
  Hopf_oscillator (leg#4) : Subsystem
  Mux1 : Mux
  Mux2 : Mux
  Scope{,3..5} (4 alike) : Scope  NumInputPorts=2
  Scope1 : Scope
  Subsystem : Subsystem
  Variable Time Delay3 : VariableTransportDelay  MaximumDelay=10  MaximumPoints=4096  ZeroDelay=on
  alpha_r_vec : Constant  Value=zeros(4,1)
  amplitude of steady-state oscillation : Constant  Value=A
  coupling oscillators : Constant  Value=phi_vec
  coupling strength : Constant  Value=epsilon
  diff. phase between zlpha_b and z_l : Constant  Value=z_l_diff
  leg_coupling : MATLAB Function  TreatAsAtomicUnit=on
  oscillation frequency : Constant  Value=f
  regulate speed of convergence : Constant  Value=k
  shape ratio of rising phase : Constant  Value=alpha
  speed of phase switching : Constant  Value=tau
  Out2 : Outport
  wires:
  [k] -> Hopf_oscillator (leg#4)/1(k)
  [tau] -> Hopf_oscillator (leg#3)/5(tau)
  [u4] -> Mux2/4
  [v2] -> Mux1/2
  shape ratio of rising phase/1 -> [alpha]
  [epsilon] -> leg_coupling/1(epsilon)
  [u3] -> Mux2/3
  [v_vec] -> leg_coupling/3(v_vec)
  [C2] -> Hopf_oscillator (leg#2)/6(C)
  leg_coupling/4(C_leg4) -> [C4]
  [f] -> Hopf_oscillator (leg#3)/3(f)
  Hopf_oscillator (leg#4)/1(u) -> [u4], Scope5/1  "theta4"
  Hopf_oscillator (leg#4)/2(v) -> [v4], Scope5/2  "latent variable"
  [k] -> Hopf_oscillator (leg#3)/1(k)
  leg_coupling/2(C_leg2) -> [C2]
  oscillation frequency/1 -> [f]
  [u1] -> Mux2/1
  Hopf_oscillator (leg#3)/1(u) -> [u3], Scope4/1  "theta3"
  [A] -> Hopf_oscillator (leg#3)/2(A)
  leg_coupling/3(C_leg3) -> [C3]
  [u2] -> Mux2/2
  Hopf_oscillator (leg#1)/2(v) -> [v1], Scope/2  "latent variable"
  [alpha] -> Hopf_oscillator (leg#2)/4(alpha)
  Hopf_oscillator (leg#3)/2(v) -> [v3], Scope4/2  "latent variable"
  speed of phase switching/1 -> [tau]
  [f] -> Hopf_oscillator (leg#2)/3(f)
  [tau] -> Hopf_oscillator (leg#4)/5(tau)
  [u_vec] -> leg_coupling/2(u_vec)
  [alpha] -> Hopf_oscillator (leg#3)/4(alpha)
  amplitude of steady-state oscillation/1 -> [A]
  [A] -> Hopf_oscillator (leg#1)/2(A)
  [A] -> Hopf_oscillator (leg#2)/2(A)
  leg_coupling/1(C_leg1) -> [C1]
  Mux2/1 -> [u_vec], [alpha_b_vec], Scope1/1
  Hopf_oscillator (leg#2)/1(u) -> [u2], Scope3/1  "theta2"
  [v4] -> Mux1/4
  [f] -> Hopf_oscillator (leg#4)/3(f)
  [C4] -> Hopf_oscillator (leg#4)/6(C)
  [C3] -> Hopf_oscillator (leg#3)/6(C)
  [tau] -> Hopf_oscillator (leg#1)/5(tau)
  coupling strength/1 -> [epsilon]
  [A] -> Hopf_oscillator (leg#4)/2(A)
  [k] -> Hopf_oscillator (leg#2)/1(k)
  [alpha] -> Hopf_oscillator (leg#4)/4(alpha)
  [v3] -> Mux1/3
  [k] -> Hopf_oscillator (leg#1)/1(k)
  [phi_vec] -> leg_coupling/4(phi_vec)
  [C1] -> Hopf_oscillator (leg#1)/6(C)
  [v1] -> Mux1/1
  Mux1/1 -> [v_vec]
  [tau] -> Hopf_oscillator (leg#2)/5(tau)
  [f] -> Hopf_oscillator (leg#1)/3(f)
  regulate speed of convergence/1 -> [k]
  Hopf_oscillator (leg#2)/2(v) -> [v2], Scope3/2  "latent variable"
  Hopf_oscillator (leg#1)/1(u) -> [u1], Scope/1  "theta1"
  [alpha] -> Hopf_oscillator (leg#1)/4(alpha)
  coupling oscillators/1 -> [phi_vec]
  [alpha_b_vec] -> Variable Time Delay3/1
  [z_l_diff] -> Variable Time Delay3/2
  Variable Time Delay3/1 -> [z_l_vec]
  alpha_r_vec/1 -> [alpha_r_vec]
  [alpha_r_vec] -> Subsystem/1(alpha_r_vec)
  [alpha_b_vec] -> Subsystem/2(alpha_b_vec)
  [z_l_vec] -> Subsystem/3(z_l_vec)
  Subsystem/1(Out1) -> Out2/1
  diff. phase between zlpha_b and z_l/1 -> [z_l_diff]

== system energy_rigid_wireOnly_quadruped_CPG_BO_fh/Act2Angle/Human expert ==
  Constant : Constant  Value=phase_delay(1)*0+0.4  SampleTime=Ts
  Constant1 : Constant  Value=phase_delay(2)*0  SampleTime=Ts
  Constant2 : Constant  Value=phase_delay(3)*0+0.4  SampleTime=Ts
  Mux1 : Mux  Inputs=3
  Mux2 : Mux
  Mux3 : Mux  Commented=on  Inputs=3
  Sine Wave : Sin  Frequency=2*pi/0.8  SampleTime=Ts
  Sine Wave1 : Sin  Frequency=2*pi/0.8  Phase=pi  SampleTime=Ts
  Variable Time Delay : VariableTransportDelay  MaximumDelay=10  MaximumPoints=4096  ZeroDelay=on
  Variable Time Delay1 : VariableTransportDelay  MaximumDelay=10  MaximumPoints=4096  ZeroDelay=on
  Variable Time Delay2 : VariableTransportDelay  MaximumDelay=10  MaximumPoints=4096  ZeroDelay=on
  alpha_b : simulink/Sources/Repeating Sequence  Commented=on  rep_seq_t=[0 0.2 0.4 0.6 0.8]  rep_seq_y=[0 1 0 -1 0]
  alpha_b1 : simulink/Sources/Repeating Sequence  Commented=on  rep_seq_t=[0 0.2 0.4 0.6 0.8]  rep_seq_y=[0 -1 0 1 0]
  alpha_r : Constant  Value=0
  alpha_r1 : Constant  Commented=on  Value=0
  z_l : simulink/Sources/Repeating Sequence  Commented=on  rep_seq_t=[0 0.2 0.4 0.6 0.8]  rep_seq_y=[-1 1 1 1 -1]
  z_l1 : simulink/Sources/Repeating Sequence  Commented=on  rep_seq_t=[0 0.2 0.4 0.6 0.8]  rep_seq_y=[1 1 -1 1 1]
  Out1 : Outport
  wires:
  Mux2/1 -> Out1/1
  Mux1/1 -> Variable Time Delay2/1, Variable Time Delay/1, Mux2/1, Variable Time Delay1/1
  Sine Wave/1 -> Mux1/2  "alpha_b_Ref"
  alpha_r/1 -> Mux1/1  "alpha_r_Ref"
  Sine Wave1/1 -> Mux1/3  "z_l_Ref"
  Constant/1 -> Variable Time Delay/2
  z_l1/1 -> Mux3/3  "z_l_Ref"
  alpha_r1/1 -> Mux3/1  "alpha_r_Ref"
  alpha_b1/1 -> Mux3/2  "alpha_b_Ref"
  Variable Time Delay/1 -> Mux2/2
  Constant1/1 -> Variable Time Delay1/2
  Variable Time Delay2/1 -> Mux2/4
  Variable Time Delay1/1 -> Mux2/3
  Constant2/1 -> Variable Time Delay2/2

== system energy_rigid_wireOnly_quadruped_CPG_BO_fh/Act2Angle/Subsystem ==
  Acts : Inport
  Demux : Demux
  FL : Subsystem
  FR : Subsystem
  Mux : Mux
  RL : Subsystem
  RR : Subsystem
  refs : Outport
  wires:
  Demux/4 -> RR/1(act)
  FR/1(angle) -> Mux/1
  Demux/2 -> FL/1(act)
  RL/1(angle) -> Mux/3
  Demux/3 -> RL/1(act)
  Demux/1 -> FR/1(act)
  RR/1(angle) -> Mux/4
  FL/1(angle) -> Mux/2
  Acts/1 -> Demux/1
  Mux/1 -> refs/1
